simulink model "RedCrane_Control_System_17032025"  (R2024b)
settings: Solver=VariableStepAuto  StartTime=0.0  StopTime=44  RelTol=1e-8
model workspace (MATLAB code in the model file):
  | %% Geometric properties
  | 
  | %Basic geometry width
  | w0 = 0.07;
  | w1 = w0/4;
  | l_RJ = 0.277; %2.1*w0;
  | r_RJ = 0.030;
  | 
  | %Column geometry
  | L_Column = 1.5655; %2;
  | eta_B = -0.25;
  | zeta_B = L_Column;
  | eta_D = -0.365; %0.25;
  | zeta_D = 1.4805; %1.5;
  | eta_J = 0.200; % 0.25;
  | zeta_J = 0.1195; %0.25;
  | 
  | %Column - Main boom link
  | l_DE = 0.490; % 0.5;
  | l_FE = 0.170; % 0.4;
  | 
  | %Main boom geometry
  | L_Mboom = 2.400; % 2;
  | eta_C = 2.400; % 2;
  | zeta_C = 0.070; % 0.25;
  | eta_F = 0.340; % 0.6;
  | zeta_F = 0.010; % -0.25;
  | eta_G = 2.365; % 1.75;
  | zeta_G = 0.235; % -0.25;
  | eta_K = 0.750; % 1;
  | zeta_K = 0.045; % -0.25;
  | 
  | %Main boom-Jib boom link
  | l_GH = 0.490; % 0.5;
  | l_IH = 0.220; % 0.4;
  | 
  | %Jib boom geometry
  | L_Jib_boom = 2.429; % 2;
  | eta_I = 0.280; % 0.5;
  | zeta_I = 0.005; % -0.25;
  | eta_TP = L_Jib_boom;
  | zeta_TP = 0;
  | 
  | % Winch
  | r_W = 0.205/2;
  | L_W = 0.191;
  | eta_W = 0.28722;
  | zeta_W = -0.29926;
  | beta_W = -0.335;
  | 
  | % Mounting plate
  | eta_MP = -0.0249;
  | zeta_MP = -0.17479;
  | beta_MP = 0;
  | 
  | % Pulley
  | r_P = 0.210/2; % Radius pulley
  | eta_P = 2.140;
  | zeta_P = -0.0506;
  | beta_P = -0.0;
  | 
  | %Roller
  | r_RO = 0.055/2; % Radius roller over
  | r_RU = 0.046/2; % Radius roller under
  | eta_RO = 0.306;
  | zeta_RO = 0.12510;
  | 
  | %Mounting
  | L_M = 1; %m
  | W_M = 1; %m
  | H_M = 1; %m
  | eta_M = 0; %m
  | zeta_M = -0.5; %m
  | beta_M = 0; %m
  | 
  | %Ground
  | L_ground = 6; %m
  | W_ground = 4; %m
  | H_ground = 0.01; %m
  | eta_ground = 1.5; %m
  | zeta_ground = -0.5; %m
  | beta_ground = 0; %m
  | 
  | 
  | %% Mass properties (Mass and center of mass)
  | column_mass = 239.4; % kg
  | column_COM = [-0.1007, 0.0001, 0.4351]; % m
  | 
  | MainBoom_mass = 216.5; % kg
  | MainBoom_COM = [1.134, 0.1674, -0.0018]; % m
  | 
  | JibBoom_mass = 842.2; % kg
  | JibBoom_COM = [0.9806, 0.1814, -0.2939]; % m
  | 
  | % Dogbone
  | E2F_mass = 7.076*2; % kg
  | E2F_COM = [0.0817, 0, 0]; % m
  | 
  | D2E_mass = 6.426*2; % kg
  | D2E_COM = [0.245, 0, 0]; % m
  | 
  | G2H_mass = 6.426*2; % kg
  | G2H_COM = [0.245, 0, 0]; % m
  | 
  | H2I_mass = 22.05; % kg
  | H2I_COM = [0.1206, 0, 0]; % m
  | 
  | % Main cylinder
  | MainC_bottom_mass = 57.9561; % kg
  | MainC_bottom_COM = [0.0081, -0.001, 0.4125]; % m
  | 
  | MainC_rod_mass = 43.93; % kg
  | MainC_rod_COM = [0, 0, -0.4290]; % m
  | 
  | % Jib cylinder
  | JibC_bottom_mass = 55.7738; % kg
  | JibC_bottom_COM = [0.0038, 0.0022, 0.4468]; % m
  | 
  | JibC_rod_mass = 45.8854; % kg
  | JibC_rod_COM = [0, 0, -0.4694]; % m
  | 
  | % Winch
  | Winch_mass = 54; % kg
  | Winch_COM = [0, 0, 0]; % m
  | 
  | 
  | %% Inertia properties (Moments of inertia and products of inertia)
  | 
  | column_MOI = [109, 114, 9.009]; % kg*m^2
  | column_POI = [0.0319, -21.59, -0.0113]; % kg*m^2
  | 
  | MainBoom_MOI = [6.5, 160.3, 160]; % kg*m^2
  | MainBoom_POI = [0.0666, 0.1093, 8.016]; % kg*m^2
  | 
  | JibBoom_MOI = [31.75, 566.3, 573.1]; % kg*m^2
  | JibBoom_POI = [-0.0237, -11.42, 9.588]; % kg*m^2
  | 
  | % Dogbone
  | E2F_MOI = [0.0111, 0.0546, 0.0587]; % kg*m^2
  | E2F_POI = [0, -0.0089, 0]; % kg*m^2
  | 
  | D2E_MOI = [0.0069, 0.2419, 0.2485]; % kg*m^2
  | D2E_POI = [0, 0, 0]; % kg*m^2
  | 
  | G2H_MOI = [0.0069, 0.2419, 0.2485]; % kg*m^2
  | G2H_POI = [0, 0, 0]; % kg*m^2
  | 
  | H2I_MOI = [0.2636, 0.4184, 0.1901]; % kg*m^2
  | H2I_POI = [0, 0, 0]; % kg*m^2
  | 
  | 
  | % Main cylinder
  | MainC_bottom_MOI = [7.2059, 7.2304, 0.3979]; % kg*m^2
  | MainC_bottom_POI = [-0.0126, -0.1802, 0.0002]; % kg*m^2
  | 
  | MainC_rod_MOI = [6.0014, 5.9633, 0.1401]; % kg*m^2
  | MainC_rod_POI = [0, -0.0001, 0]; % kg*m^2
  | 
  | % Jib cylinder
  | JibC_bottom_MOI = [8.3780, 8.3476, 0.3607]; % kg*m^2
  | JibC_bottom_POI = [-0.0119, -0.1037, 0.0033]; % kg*m^2
  | 
  | JibC_rod_MOI = [7.4245, 7.3864, 0.1401]; % kg*m^2
  | JibC_rod_POI = [0, -0.0001, 0]; % kg*m^2
  | 
  | % Winch
  | I_W_xx = (1/4)*Winch_mass*r_W^2 + (1/12)*Winch_mass*L_W^2;
  | I_W_yy = (1/4)*Winch_mass*r_W^2 + (1/12)*Winch_mass*L_W^2;
  | I_W_zz = (1/2)*Winch_mass*r_W^2;
  | 
  | Winch_MOI = [I_W_xx, I_W_yy, I_W_zz]; % kg*m^2
  | Winch_POI = [0, 0, 0]; % kg*m^2
  | 
  | 
  | %% Hydraulics
  | 
  | %-------------Cylinder---------------------
  | 
  | % Main cylinder
  | D_piston_MainC = 160; %mm dimater of piston side
  | L_piston_MainC = 65; %66.2;%mm length from joint to buttom of piston side
  | D_rod_MainC = 100; %mm diamter of cylinder rod
  | L_rod_MainC = 978; %990;%mm length from bottom of rod to joint
  | A_piston_MainC = pi/4*D_piston_MainC^2; % mm^2 area of piston side
  | A_rod_MainC = pi/4*D_rod_MainC^2; % mm^2 area of rod
  | A_rodside_MainC = A_piston_MainC-A_rod_MainC; % mm^2 area of rod side
  | L_barrel_MainC = 945-L_piston_MainC; %mm
  | stroke_MainC = 0.75; %m
  | initial_pos_Main = 0.3; %m
  | initial_Pa_Main = 17;%Bar
  | 
  | % Jib cylinder
  | D_piston_JibC = 150; %mm dimater of piston side
  | L_piston_JibC = 65; %66.2;%mm length from joint to buttom of piston side
  | D_rod_JibC = 100; %mm diamter of cylinder rod
  | L_rod_JibC = 1089.5; %1105.5;%mm length from bottom of rod to joint
  | A_piston_JibC = pi/4*D_piston_JibC^2; % mm^2 area of piston side
  | A_rod_JibC = pi/4*D_rod_JibC^2; % mm^2 area of rod
  | A_rodside_JibC = A_piston_JibC-A_rod_JibC; % mm^2 area of rod side
  | L_barrel_JibC = 1050-L_piston_JibC; %mm
  | stroke_JibC = 0.855; %m
  | initial_pos_Jib = 0.855; %m
  | initial_Pa_Jib = 1;%Bar
  | initial_Pb_Jib = 67;%Bar
  | 
  | % winch
  | poly_b = [1.762740809095876e+02,-44.442169999547330];
  | poly_c = [1.901177983521692e+02,-1.484122102902541e+02];
  | angle_b = poly_b(1)*initial_pos_Main + poly_b(2);
  | angle_c = poly_c(1)*initial_pos_Jib + poly_c(2);
  | angle_w = -90 - angle_c - angle_b;
  | 
  | %Motor
  | DM = 200; %Displacement cm^3/rev
  | GR = 5.04; % Gear ratio 1:5,04
  | 
  | 
  | % ------------------CBV-------------------
  | 
  | % Main
  | pCr_Main = 43.95;%Bar
  | dp_open_Main = 124.43;%Bar
  | 
  | % Jib
  | alpha = 2.7;
  | pCr_Jib_A = 320;%Bar
  | dp_open_Jib_A = 65;%Bar
  | pCr_Jib_B = 280;%Bar
  | dp_open_Jib_B = 40;%Bar
  | 
  | %-------------------DCV-----------------------
  | Cd = 0.64;
  | Q_rat = 30/6e4;
  | dp_2 = 6e5;
  | dp_1 = 1e5;
  | roh = 850;
  | 
  | % Main dcv
  | dead_up_Main = 0.071;
  | dead_down_Main = 0.126;
  | 
  | % Jib dcv
  | dead_up_Jib = 0.037;
  | dead_down_Jib = 0.126;
  | 
  | Ad2 = Q_rat/(Cd*sqrt(2/roh*dp_2))*1e6; %mm
  | Ad1_1 = Q_rat/(Cd*sqrt(2/roh*dp_1))*1e6;
  | Ad1_0 = Q_rat/(Cd*sqrt(2/roh*dp_1))*1e6*0;
  | 
  | Ad1_Main_up = Q_rat/(Cd*sqrt(2/roh*dp_1))*1e6*dead_up_Main;
  | Ad1_Main_down = Q_rat/(Cd*sqrt(2/roh*dp_1))*1e6*dead_down_Main;
  | Ad1_Jib_up = Q_rat/(Cd*sqrt(2/roh*dp_1))*1e6*dead_up_Jib;
  | Ad1_Jib_down = Q_rat/(Cd*sqrt(2/roh*dp_1))*1e6*dead_down_Jib;
undefined symbols (not defined in the file or in its folder): dead_down_m, dead_up_m, X, Y, Z
libraries: sm_lib x171, fl_lib x94, nesl_utility x64, SimscapeFluids_lib x33, sdl_lib x1
(part 5 of 9)

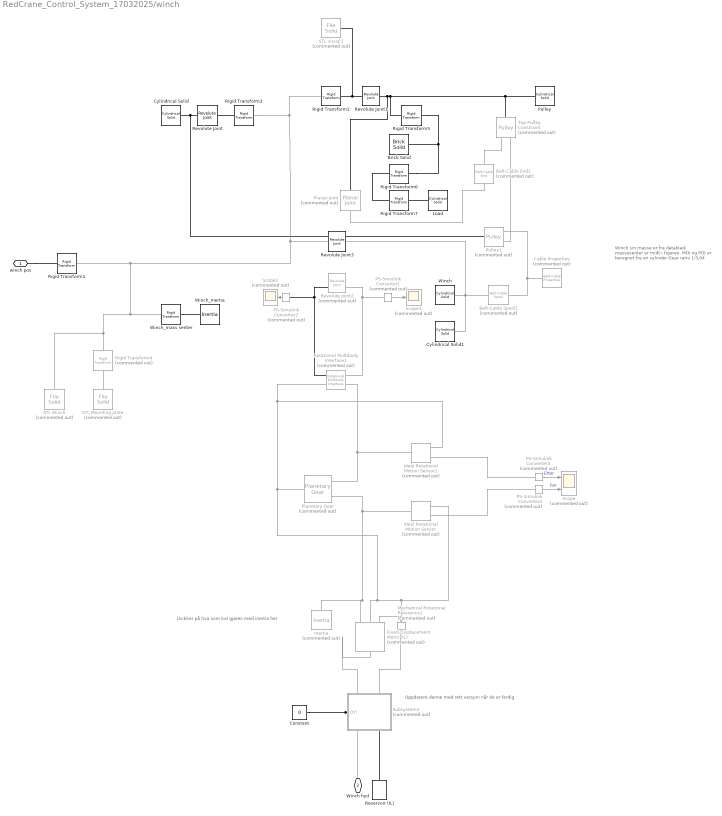
== system RedCrane_Control_System_17032025/winch ==
  note: Oppdatere denne med rett versjon når de er
      | ferdig
  note: Winch sin masse er fra datablad,
      | massesenter er midt i figuren.
      |
      | MOI og POI er beregnet fra en
      | sylinder
      |
      | Gear ratio 1:5,04
  note: Usikker på hva som kal gjøres med inertia her
  Belt-Cable End2 : sm_lib/Belts and Cables/Belt-Cable End  Commented=on
  Belt-Cable Spool1 : sm_lib/Belts and Cables/Belt-Cable Spool  Commented=on  PitchRadius=r_W  PitchRadiusUnits=m  SenseSpoolAngleA=off  SenseFleetAngleA=off
  Brick Solid : sm_lib/Body Elements/Brick Solid  BrickDimensions=[1 0.01 0.01]  BrickDimensionsUnits=m  ExportEntireGeometry=off  InertiaType=CalculateFromGeometry  BasedOnType=Density  Density=0  DensityUnits=kg/m^3  Mass=1  MassUnits=kg  CenterOfMass=[0 0 0]  CenterOfMassUnits=m  MomentsOfInertia=[1 1 1]  MomentsOfInertiaUnits=kg*m^2  ProductsOfInertia=[0 0 0]  ProductsOfInertiaUnits=kg*m^2  GraphicType=FromGeometry  MarkerShape=Sphere  MarkerSize=10  GraphicVisPropType=SimpleVisualProperties  GraphicDiffuseColor=[0.5 0.5 0.5]  GraphicOpacity=1  GraphicSpecularColor=[0.5 0.5 0.5 1.0]  GraphicAmbientColor=[0.15 0.15 0.15 1.0]  GraphicEmissiveColor=[0.0 0.0 0.0 1.0]  GraphicShininess=75  DoExposeReferenceFrame=on  SerializedFrames=<Frames/>
  Cable Properties : sm_lib/Belts and Cables/Belt-Cable Properties  Commented=on  DrumBeltCableAlignment=Unrestricted  GraphicType=PitchLine  GraphicVisPropType=SimpleVisualProperties  GraphicDiffuseColor=[0.4 0.0 1.0]  GraphicOpacity=1.0  GraphicSpecularColor=[0.5 0.5 0.5 1.0]  GraphicAmbientColor=[0.15 0.15 0.15 1.0]  GraphicEmissiveColor=[0.0 0.0 0.0 1.0]  GraphicShininess=75
  Constant : Constant  Value=0
  Cylindrical Solid : sm_lib/Body Elements/Cylindrical Solid  CylinderRadius=r_RO  CylinderRadiusUnits=m  CylinderLength=L_W  CylinderLengthUnits=m  ExportEntireGeometry=off  InertiaType=Custom  BasedOnType=Density  Density=1000  DensityUnits=kg/m^3  Mass=1  MassUnits=kg  CenterOfMass=[0 0 0]  CenterOfMassUnits=m  MomentsOfInertia=[1 1 1]  MomentsOfInertiaUnits=kg*m^2  ProductsOfInertia=[0 0 0]  ProductsOfInertiaUnits=kg*m^2  GraphicType=FromGeometry  MarkerShape=Sphere  MarkerSize=10  GraphicVisPropType=SimpleVisualProperties  GraphicDiffuseColor=[1 1 1]  GraphicOpacity=1  GraphicSpecularColor=[0.5 0.5 0.5 1.0]  GraphicAmbientColor=[0.15 0.15 0.15 1.0]  GraphicEmissiveColor=[0.0 0.0 0.0 1.0]  GraphicShininess=75  DoExposeReferenceFrame=on  SerializedFrames=<Frames/>
  Cylindrical Solid1 : sm_lib/Body Elements/Cylindrical Solid  CylinderRadius=(305-10.5)/2  CylinderRadiusUnits=mm  CylinderLength=0.2  CylinderLengthUnits=m  ExportEntireGeometry=off  InertiaType=PointMass  BasedOnType=Density  Density=1000  DensityUnits=kg/m^3  Mass=279.7880-50  MassUnits=kg  CenterOfMass=[0 0 0]  CenterOfMassUnits=m  MomentsOfInertia=[1 1 1]  MomentsOfInertiaUnits=kg*m^2  ProductsOfInertia=[0 0 0]  ProductsOfInertiaUnits=kg*m^2  GraphicType=FromGeometry  MarkerShape=Sphere  MarkerSize=10  GraphicVisPropType=SimpleVisualProperties  GraphicDiffuseColor=[0.902 0.902 0.902]  GraphicOpacity=1  GraphicSpecularColor=[0.5 0.5 0.5 1.0]  GraphicAmbientColor=[0.15 0.15 0.15 1.0]  GraphicEmissiveColor=[0.0 0.0 0.0 1.0]  GraphicShininess=75  DoExposeReferenceFrame=on  SerializedFrames=<Frames/>
  Fixed-Displacement Motor (IL) : SimscapeFluids_lib/Isothermal Liquid/Pumps & Motors/Fixed-Displacement Motor (IL)  Commented=on  leakage_friction_spec=fluids.isothermal_liquid.pumps_motors.enum.MotorLossSpec.Analytical  displacement=DM cm^3/rev  omega_nominal=1800 rpm  p_nominal=10 MPa  vol_eff_nominal=1  mech_eff_nominal=1  no_load_torque=0 N*m  p_diff_eff_TLU=[.1, 1, 2] MPa  omega_eff_TLU=[250, 500, 1000, 2000, 3000, 4000] rpm  vol_eff_TLU=[.816, .908, .954, .977, .981, .984; .325, .663, .831, .916, .925, .946; .137, .568, .78, .892, .893, .91]  mech_eff_TLU=[.996, .996, .996, .996, .996, .996; .988, .989, .989, .989, .989, .99; .981, .981, .982, .982, .983, .984]  p_diff_loss_TLU=[.1, 1, 2] MPa  omega_loss_TLU=[250, 500, 1000, 2000, 3000, 4000] rpm  vol_loss_TLU=1e-3 * [.023, .023, .023, .023, .0285, .032; .0844, .0842, .0845, .084, .1125, .108; .1079, .108, .11, .108, .1605, .18] m^3/s  mech_loss_TLU=[.002, .002, .002, .002, .002, .002; .0607, .0556, .0556, .0556, .0556, .0505; .1937, .1937, .1833, .1833, .1729, .1626] N*m  q_shaft_TLU=[.125, .25, .5, 1, 1.5, 2] * 1e-3 m^3/s  p_diff_shaft_TLU=[.1, 1, 2] MPa  torque_shaft_TLU=[.47, 4.72, 9.35; .47, 4.7, 9.36; .47, 4.7, 9.4; .47, 4.7, 9.41; .47, 4.7, 9.46; .47, 4.68, 9.5] N*m  omega_shaft_TLU=[205, 80, 35; 455, 330, 285; 955, 831, 780; 1950, 1830, 1780; 2940, 2775, 2680; 3940, 3780, 3640] rpm  vol_eff_min=1e-3  vol_eff_max=1  mech_eff_min=1e-3  mech_eff_max=1  pressure_threshold=1e-3 MPa  omega_threshold=100 rpm  supplied_range_check=simscape.enum.assert.action.none  motor_mode_check=simscape.enum.assert.action.none  pressure_check=simscape.enum.assert.action.none  p_min_valid=0.101325 MPa
      settings: InternalSimscapePortConfiguration="{\"Bottom\":[{\"id\":\"B\",\"label\":\"B\",\"type\":\"foundation.isothermal_liquid.isothermal_liquid\"}],\"Left\":[],\"Right\":[{\"id\":\"R\",\"label\":\"R\",\"type\":\"foundation.mechanical.rotational.rotational\"},{\"id\":\"C\",\"label\":\"C\",\"type\":\"foundation.mechanical.rotational.rotational\"}],\"Top\":[{\"id\":\"A\",\"label\":\"A\",\"type\":\"foundation.isothermal_liquid.isothermal_liquid\"}]}"
  Ideal Rotational Motion Sensor : fl_lib/Mechanical/Mechanical Sensors/Ideal Rotational Motion Sensor  Commented=on  reference=foundation.enum.MeasurementReference.difference  acceleration_port=false  velocity_port=true  position_port=false  wrap_angle=false  offset=0 rad
      settings: InternalSimscapePortConfiguration="{\"Bottom\":[],\"Left\":[{\"id\":\"R\",\"label\":\"R\",\"type\":\"foundation.mechanical.rotational.rotational\"}],\"Right\":[{\"id\":\"C\",\"label\":\"C\",\"type\":\"foundation.mechanical.rotational.rotational\"},{\"id\":\"W\",\"label\":\"W\",\"type\":\"output\"}],\"Top\":[]}"
  Ideal Rotational Motion Sensor1 : fl_lib/Mechanical/Mechanical Sensors/Ideal Rotational Motion Sensor  Commented=on  reference=foundation.enum.MeasurementReference.difference  acceleration_port=false  velocity_port=true  position_port=false  wrap_angle=false  offset=0 rad
      settings: InternalSimscapePortConfiguration="{\"Bottom\":[],\"Left\":[{\"id\":\"R\",\"label\":\"R\",\"type\":\"foundation.mechanical.rotational.rotational\"}],\"Right\":[{\"id\":\"C\",\"label\":\"C\",\"type\":\"foundation.mechanical.rotational.rotational\"},{\"id\":\"W\",\"label\":\"W\",\"type\":\"output\"}],\"Top\":[]}"
  Inertia : fl_lib/Mechanical/Rotational Elements/Inertia  Commented=on  inertia=0.01 kg*m^2  num_ports=foundation.enum.numPorts2.one  w_specify=off  w_priority=High  w=0 rad/s  w_nominal_specify=off  w_nominal_value=1  w_nominal_unit=rad/s  t_specify=off  t_priority=None  t=0 N*m  t_nominal_specify=off  t_nominal_value=1  t_nominal_unit=N*m
  Load : sm_lib/Body Elements/Cylindrical Solid  CylinderRadius=81/2  CylinderRadiusUnits=mm  CylinderLength=240  CylinderLengthUnits=mm  ExportEntireGeometry=off  InertiaType=CalculateFromGeometry  BasedOnType=Mass  Density=1000  DensityUnits=kg/m^3  Mass=10  MassUnits=kg  CenterOfMass=[0 0 0]  CenterOfMassUnits=m  MomentsOfInertia=[1 1 1]  MomentsOfInertiaUnits=kg*m^2  ProductsOfInertia=[0 0 0]  ProductsOfInertiaUnits=kg*m^2  GraphicType=FromGeometry  MarkerShape=Sphere  MarkerSize=10  GraphicVisPropType=SimpleVisualProperties  GraphicDiffuseColor=[0.9412 0.9412 0.07451]  GraphicOpacity=1  GraphicSpecularColor=[0.5 0.5 0.5 1.0]  GraphicAmbientColor=[0.15 0.15 0.15 1.0]  GraphicEmissiveColor=[0.0 0.0 0.0 1.0]  GraphicShininess=75  DoExposeReferenceFrame=on  SerializedFrames=<Frames/>
  Mechanical Rotational Reference1 : fl_lib/Mechanical/Rotational Elements/Mechanical Rotational Reference  Commented=on
  PS-Simulink Converter{1..4} (4 alike) : nesl_utility/PS-Simulink Converter  Commented=on  PhysicalDomain=network_engine_domain  SubClassName=ps_output  LeftPortType=input  RightPortType=output  PseudoPeriodic=off  Frequencies=[]  VectorFormat=inherit  Unit=inherit  AffineConversion=off
  Planar Joint : sm_lib/Joints/Planar Joint  Commented=on  JointMode=Normal  CompositeWrenchDir=FollowerOnBase  CompositeWrenchFrame=BaseFrame  SenseConstraintForce=off  SenseConstraintTorque=off  SenseTotalForce=off  SenseTotalTorque=off  PxPositionTargetSpecify=on  PxPositionTargetPriority=High  PxPositionTargetValue=1  PxPositionTargetValueUnits=m  PxVelocityTargetSpecify=off  PxVelocityTargetPriority=High  PxVelocityTargetValue=0  PxVelocityTargetValueUnits=m/s  PxEquilibriumPosition=0  PxEquilibriumPositionUnits=m  PxSpringStiffness=0  PxSpringStiffnessUnits=N/m  PxDampingCoefficient=1e-1  PxDampingCoefficientUnits=N/(m/s)  PxLowerLimitSpecify=off  PxLowerLimitBound=-1  PxLowerLimitBoundUnits=m  PxLowerLimitStiffness=1e6  PxLowerLimitStiffnessUnits=N/m  PxLowerLimitDamping=1e3  PxLowerLimitDampingUnits=N/(m/s)  PxLowerLimitTransitionRegionWidth=1e-4  PxLowerLimitTransitionRegionWidthUnits=m  PxUpperLimitSpecify=off  PxUpperLimitBound=1  PxUpperLimitBoundUnits=m  PxUpperLimitStiffness=1e6  PxUpperLimitStiffnessUnits=N/m  PxUpperLimitDamping=1e3  PxUpperLimitDampingUnits=N/(m/s)  PxUpperLimitTransitionRegionWidth=1e-4  PxUpperLimitTransitionRegionWidthUnits=m  PxTorqueActuationMode=NoTorque  PxMotionActuationMode=ComputedMotion  PxSensePosition=off  PxSenseVelocity=off  PxSenseAcceleration=off  PxSenseTorqueForce=off  PxSenseLowerLimitTorqueForce=off  PxSenseUpperLimitTorqueForce=off  PyPositionTargetSpecify=on  PyPositionTargetPriority=High  PyPositionTargetValue=r_P  PyPositionTargetValueUnits=m  PyVelocityTargetSpecify=off  PyVelocityTargetPriority=High  PyVelocityTargetValue=0  PyVelocityTargetValueUnits=m/s  PyEquilibriumPosition=0  PyEquilibriumPositionUnits=m  PySpringStiffness=0  PySpringStiffnessUnits=N/m  PyDampingCoefficient=1e-1  PyDampingCoefficientUnits=N/(m/s)  PyLowerLimitSpecify=off  PyLowerLimitBound=-1  PyLowerLimitBoundUnits=m  PyLowerLimitStiffness=1e6  PyLowerLimitStiffnessUnits=N/m  PyLowerLimitDamping=1e3  PyLowerLimitDampingUnits=N/(m/s)  PyLowerLimitTransitionRegionWidth=1e-4  PyLowerLimitTransitionRegionWidthUnits=m  PyUpperLimitSpecify=off  PyUpperLimitBound=1  PyUpperLimitBoundUnits=m  PyUpperLimitStiffness=1e6  PyUpperLimitStiffnessUnits=N/m  PyUpperLimitDamping=1e3  PyUpperLimitDampingUnits=N/(m/s)  PyUpperLimitTransitionRegionWidth=1e-4  PyUpperLimitTransitionRegionWidthUnits=m  PyTorqueActuationMode=NoTorque  PyMotionActuationMode=ComputedMotion  PySensePosition=off  PySenseVelocity=off  PySenseAcceleration=off  PySenseTorqueForce=off  PySenseLowerLimitTorqueForce=off  PySenseUpperLimitTorqueForce=off  RzPositionTargetSpecify=off  RzPositionTargetPriority=High  RzPositionTargetValue=90  RzPositionTargetValueUnits=deg  RzVelocityTargetSpecify=off  RzVelocityTargetPriority=High  RzVelocityTargetValue=0  RzVelocityTargetValueUnits=deg/s  RzEquilibriumPosition=0  RzEquilibriumPositionUnits=deg  RzSpringStiffness=0  RzSpringStiffnessUnits=N*m/deg  RzDampingCoefficient=0  RzDampingCoefficientUnits=N*m/(deg/s)  RzLowerLimitSpecify=off  RzLowerLimitBound=-90  RzLowerLimitBoundUnits=deg  RzLowerLimitStiffness=1e4  RzLowerLimitStiffnessUnits=N*m/deg  RzLowerLimitDamping=10  RzLowerLimitDampingUnits=N*m/(deg/s)  RzLowerLimitTransitionRegionWidth=0.1  RzLowerLimitTransitionRegionWidthUnits=deg  RzUpperLimitSpecify=off  RzUpperLimitBound=90  RzUpperLimitBoundUnits=deg  RzUpperLimitStiffness=1e4  RzUpperLimitStiffnessUnits=N*m/deg  RzUpperLimitDamping=10  RzUpperLimitDampingUnits=N*m/(deg/s)  RzUpperLimitTransitionRegionWidth=0.1  RzUpperLimitTransitionRegionWidthUnits=deg  RzTorqueActuationMode=NoTorque  RzMotionActuationMode=ComputedMotion  RzSensePosition=off  RzSenseVelocity=off  RzSenseAcceleration=off  RzSenseTorqueForce=off  RzSenseLowerLimitTorqueForce=off  RzSenseUpperLimitTorqueForce=off
  Planetary Gear : sdl_lib/Gears/Planetary Gear  Commented=on  rs_ratio=GR  friction_model=sdl.enum.gear_friction.none  efficiency=[.96, .98]  temperature_TLU=[280, 300, 320] K  efficiency_sp_TLU=[.95, .9, .85]  efficiency_rp_TLU=[.95, .9, .85]  pwr_thr=[.001, .001] W  mu_visc=[0, 0] N*m*s/rad  model_inertia=simscape.enum.onoff.off  sun_inertia=0.001 kg*m^2  ring_inertia=0.001 kg*m^2  carrier_inertia=0.001 kg*m^2  carrier_radius=0.01 m  planet_inertia=0.001 kg*m^2  planet_mass=0.001 kg  thermal_mass=50 J/K  T_init=300 K
  Pulley : sm_lib/Body Elements/Cylindrical Solid  CylinderRadius=r_P  CylinderRadiusUnits=m  CylinderLength=L_W  CylinderLengthUnits=m  ExportEntireGeometry=off  InertiaType=Custom  BasedOnType=Density  Density=1000  DensityUnits=kg/m^3  Mass=1  MassUnits=kg  CenterOfMass=[0 0 0]  CenterOfMassUnits=m  MomentsOfInertia=[1 1 1]  MomentsOfInertiaUnits=kg*m^2  ProductsOfInertia=[0 0 0]  ProductsOfInertiaUnits=kg*m^2  GraphicType=FromGeometry  MarkerShape=Sphere  MarkerSize=10  GraphicVisPropType=SimpleVisualProperties  GraphicDiffuseColor=[0.149 0.149 0.149]  GraphicOpacity=1  GraphicSpecularColor=[0.5 0.5 0.5 1.0]  GraphicAmbientColor=[0.15 0.15 0.15 1.0]  GraphicEmissiveColor=[0.0 0.0 0.0 1.0]  GraphicShininess=75  DoExposeReferenceFrame=on  SerializedFrames=<Frames/>
  Pulley1 : sm_lib/Belts and Cables/Pulley  Commented=on  PitchRadius=r_RO  PitchRadiusUnits=m  InitialWrapAngleLowerBound=0  InitialWrapAngleLowerBoundUnits=deg  SenseWrapAngle=off  SensePulleyAngleA=off  SensePulleyAngleB=off  SenseFleetAngleA=off  SenseFleetAngleB=off
  Reservoir (IL) : fl_lib/Isothermal Liquid/Elements/Reservoir (IL)  reservoir_type=foundation.enum.constant_controlled.constant  pressure_spec=foundation.enum.pressure_spec.atmospheric  reservoir_pressure=0.101325 MPa
  Revolute Joint : sm_lib/Joints/Revolute Joint  JointMode=Normal  CompositeWrenchDir=FollowerOnBase  CompositeWrenchFrame=BaseFrame  SenseConstraintForce=off  SenseConstraintTorque=off  SenseTotalForce=off  SenseTotalTorque=off  PositionTargetSpecify=off  PositionTargetPriority=High  PositionTargetValue=0  PositionTargetValueUnits=deg  VelocityTargetSpecify=off  VelocityTargetPriority=High  VelocityTargetValue=0  VelocityTargetValueUnits=deg/s  EquilibriumPosition=0  EquilibriumPositionUnits=deg  SpringStiffness=0  SpringStiffnessUnits=N*m/deg  DampingCoefficient=0  DampingCoefficientUnits=N*m/(deg/s)  LowerLimitSpecify=off  LowerLimitBound=-90  LowerLimitBoundUnits=deg  LowerLimitStiffness=1e4  LowerLimitStiffnessUnits=N*m/deg  LowerLimitDamping=10  LowerLimitDampingUnits=N*m/(deg/s)  LowerLimitTransitionRegionWidth=0.1  LowerLimitTransitionRegionWidthUnits=deg  UpperLimitSpecify=off  UpperLimitBound=90  UpperLimitBoundUnits=deg  UpperLimitStiffness=1e4  UpperLimitStiffnessUnits=N*m/deg  UpperLimitDamping=10  UpperLimitDampingUnits=N*m/(deg/s)  UpperLimitTransitionRegionWidth=0.1  UpperLimitTransitionRegionWidthUnits=deg  TorqueActuationMode=NoTorque  MotionActuationMode=ComputedMotion  SensePosition=off  SenseVelocity=off  SenseAcceleration=off  SenseTorqueForce=off  SenseLowerLimitTorqueForce=off  SenseUpperLimitTorqueForce=off
  Revolute Joint1 : sm_lib/Joints/Revolute Joint  JointMode=Normal  CompositeWrenchDir=FollowerOnBase  CompositeWrenchFrame=BaseFrame  SenseConstraintForce=off  SenseConstraintTorque=off  SenseTotalForce=off  SenseTotalTorque=off  PositionTargetSpecify=on  PositionTargetPriority=High  PositionTargetValue=angle_w  PositionTargetValueUnits=deg  VelocityTargetSpecify=on  VelocityTargetPriority=High  VelocityTargetValue=0  VelocityTargetValueUnits=deg/s  EquilibriumPosition=0  EquilibriumPositionUnits=deg  SpringStiffness=0  SpringStiffnessUnits=N*m/deg  DampingCoefficient=0  DampingCoefficientUnits=N*m/(deg/s)  LowerLimitSpecify=off  LowerLimitBound=-90  LowerLimitBoundUnits=deg  LowerLimitStiffness=1e4  LowerLimitStiffnessUnits=N*m/deg  LowerLimitDamping=10  LowerLimitDampingUnits=N*m/(deg/s)  LowerLimitTransitionRegionWidth=0.1  LowerLimitTransitionRegionWidthUnits=deg  UpperLimitSpecify=off  UpperLimitBound=90  UpperLimitBoundUnits=deg  UpperLimitStiffness=1e4  UpperLimitStiffnessUnits=N*m/deg  UpperLimitDamping=10  UpperLimitDampingUnits=N*m/(deg/s)  UpperLimitTransitionRegionWidth=0.1  UpperLimitTransitionRegionWidthUnits=deg  TorqueActuationMode=NoTorque  MotionActuationMode=ComputedMotion  SensePosition=off  SenseVelocity=off  SenseAcceleration=off  SenseTorqueForce=off  SenseLowerLimitTorqueForce=off  SenseUpperLimitTorqueForce=off
  Revolute Joint2 : sm_lib/Joints/Revolute Joint  Commented=on  JointMode=Normal  CompositeWrenchDir=FollowerOnBase  CompositeWrenchFrame=BaseFrame  SenseConstraintForce=off  SenseConstraintTorque=off  SenseTotalForce=off  SenseTotalTorque=off  PositionTargetSpecify=on  PositionTargetPriority=High  PositionTargetValue=0  PositionTargetValueUnits=deg  VelocityTargetSpecify=on  VelocityTargetPriority=High  VelocityTargetValue=0  VelocityTargetValueUnits=deg/s  EquilibriumPosition=0  EquilibriumPositionUnits=deg  SpringStiffness=0  SpringStiffnessUnits=N*m/deg  DampingCoefficient=0  DampingCoefficientUnits=N*m/(deg/s)  LowerLimitSpecify=off  LowerLimitBound=-90  LowerLimitBoundUnits=deg  LowerLimitStiffness=1e4  LowerLimitStiffnessUnits=N*m/deg  LowerLimitDamping=10  LowerLimitDampingUnits=N*m/(deg/s)  LowerLimitTransitionRegionWidth=0.1  LowerLimitTransitionRegionWidthUnits=deg  UpperLimitSpecify=off  UpperLimitBound=90  UpperLimitBoundUnits=deg  UpperLimitStiffness=1e4  UpperLimitStiffnessUnits=N*m/deg  UpperLimitDamping=10  UpperLimitDampingUnits=N*m/(deg/s)  UpperLimitTransitionRegionWidth=0.1  UpperLimitTransitionRegionWidthUnits=deg  TorqueActuationMode=InputTorque  MotionActuationMode=ComputedMotion  SensePosition=off  SenseVelocity=on  SenseAcceleration=off  SenseTorqueForce=off  SenseLowerLimitTorqueForce=off  SenseUpperLimitTorqueForce=off
  Revolute Joint3 : sm_lib/Joints/Revolute Joint  JointMode=Locked  CompositeWrenchDir=FollowerOnBase  CompositeWrenchFrame=BaseFrame  SenseConstraintForce=off  SenseConstraintTorque=off  SenseTotalForce=off  SenseTotalTorque=off  PositionTargetSpecify=on  PositionTargetPriority=High  PositionTargetValue=0  PositionTargetValueUnits=deg  VelocityTargetSpecify=on  VelocityTargetPriority=High  VelocityTargetValue=0  VelocityTargetValueUnits=deg/s  EquilibriumPosition=0  EquilibriumPositionUnits=deg  SpringStiffness=0  SpringStiffnessUnits=N*m/deg  DampingCoefficient=0  DampingCoefficientUnits=N*m/(deg/s)  LowerLimitSpecify=off  LowerLimitBound=-90  LowerLimitBoundUnits=deg  LowerLimitStiffness=1e4  LowerLimitStiffnessUnits=N*m/deg  LowerLimitDamping=10  LowerLimitDampingUnits=N*m/(deg/s)  LowerLimitTransitionRegionWidth=0.1  LowerLimitTransitionRegionWidthUnits=deg  UpperLimitSpecify=off  UpperLimitBound=90  UpperLimitBoundUnits=deg  UpperLimitStiffness=1e4  UpperLimitStiffnessUnits=N*m/deg  UpperLimitDamping=10  UpperLimitDampingUnits=N*m/(deg/s)  UpperLimitTransitionRegionWidth=0.1  UpperLimitTransitionRegionWidthUnits=deg  TorqueActuationMode=NoTorque  MotionActuationMode=ComputedMotion  SensePosition=off  SenseVelocity=off  SenseAcceleration=off  SenseTorqueForce=off  SenseLowerLimitTorqueForce=off  SenseUpperLimitTorqueForce=off
  Rigid Transform1 : sm_lib/Frames and Transforms/Rigid Transform  RotationMethod=None  FollAlignAxisA=+X  BaseAlignAxisA=+Y  FollAlignAxisB=+Y  BaseAlignAxisB=+Z  RotationStandardAxis=+Z  RotationAngle=0  RotationAngleUnits=deg  RotationArbitraryAxis=[0 0 1]  RotationSequenceAxes=FollowerAxes  RotationSequence=XYZ  RotationSequenceAngles=[90 0 0]  RotationSequenceAnglesUnits=deg  RotationMatrix=[1 0 0;0 1 0;0 0 1]  Quaternion=[1 0 0 0]  TranslationMethod=Cartesian  TranslationCartesianOffset=[eta_W zeta_W beta_W]  TranslationCartesianOffsetUnits=m  TranslationStandardAxis=+Z  TranslationStandardOffset=0  TranslationStandardOffsetUnits=m  TranslationROffset=0  TranslationROffsetUnits=m  TranslationThetaOffset=0  TranslationThetaOffsetUnits=deg  TranslationZOffset=0  TranslationZOffsetUnits=m
  Rigid Transform2 : sm_lib/Frames and Transforms/Rigid Transform  RotationMethod=None  FollAlignAxisA=+X  BaseAlignAxisA=+Y  FollAlignAxisB=+Y  BaseAlignAxisB=+Z  RotationStandardAxis=+X  RotationAngle=90  RotationAngleUnits=deg  RotationArbitraryAxis=[0 0 1]  RotationSequenceAxes=FollowerAxes  RotationSequence=XYX  RotationSequenceAngles=[0 0 0]  RotationSequenceAnglesUnits=deg  RotationMatrix=[1 0 0;0 1 0;0 0 1]  Quaternion=[1 0 0 0]  TranslationMethod=Cartesian  TranslationCartesianOffset=[eta_P zeta_P beta_P]  TranslationCartesianOffsetUnits=m  TranslationStandardAxis=+Z  TranslationStandardOffset=0  TranslationStandardOffsetUnits=m  TranslationROffset=0  TranslationROffsetUnits=m  TranslationThetaOffset=0  TranslationThetaOffsetUnits=deg  TranslationZOffset=0  TranslationZOffsetUnits=m
  Rigid Transform3 : sm_lib/Frames and Transforms/Rigid Transform  RotationMethod=None  FollAlignAxisA=+X  BaseAlignAxisA=+Y  FollAlignAxisB=+Y  BaseAlignAxisB=+Z  RotationStandardAxis=+X  RotationAngle=90  RotationAngleUnits=deg  RotationArbitraryAxis=[0 0 1]  RotationSequenceAxes=FollowerAxes  RotationSequence=XYX  RotationSequenceAngles=[0 0 0]  RotationSequenceAnglesUnits=deg  RotationMatrix=[1 0 0;0 1 0;0 0 1]  Quaternion=[1 0 0 0]  TranslationMethod=Cartesian  TranslationCartesianOffset=[eta_RO zeta_RO 0]  TranslationCartesianOffsetUnits=m  TranslationStandardAxis=+Z  TranslationStandardOffset=0  TranslationStandardOffsetUnits=m  TranslationROffset=0  TranslationROffsetUnits=m  TranslationThetaOffset=0  TranslationThetaOffsetUnits=deg  TranslationZOffset=0  TranslationZOffsetUnits=m
  Rigid Transform4 : sm_lib/Frames and Transforms/Rigid Transform  Commented=on  RotationMethod=None  FollAlignAxisA=+X  BaseAlignAxisA=+Y  FollAlignAxisB=+Y  BaseAlignAxisB=+Z  RotationStandardAxis=-X  RotationAngle=90  RotationAngleUnits=deg  RotationArbitraryAxis=[0 0 1]  RotationSequenceAxes=FollowerAxes  RotationSequence=XYX  RotationSequenceAngles=[0 0 0]  RotationSequenceAnglesUnits=deg  RotationMatrix=[1 0 0;0 1 0;0 0 1]  Quaternion=[1 0 0 0]  TranslationMethod=Cartesian  TranslationCartesianOffset=[eta_MP zeta_MP beta_MP]  TranslationCartesianOffsetUnits=m  TranslationStandardAxis=+Z  TranslationStandardOffset=0  TranslationStandardOffsetUnits=m  TranslationROffset=0  TranslationROffsetUnits=m  TranslationThetaOffset=0  TranslationThetaOffsetUnits=deg  TranslationZOffset=0  TranslationZOffsetUnits=m
  Rigid Transform5 : sm_lib/Frames and Transforms/Rigid Transform  RotationMethod=None  FollAlignAxisA=+X  BaseAlignAxisA=+Y  FollAlignAxisB=+Y  BaseAlignAxisB=+Z  RotationStandardAxis=+X  RotationAngle=90  RotationAngleUnits=deg  RotationArbitraryAxis=[0 0 1]  RotationSequenceAxes=FollowerAxes  RotationSequence=XYX  RotationSequenceAngles=[0 0 0]  RotationSequenceAnglesUnits=deg  RotationMatrix=[1 0 0;0 1 0;0 0 1]  Quaternion=[1 0 0 0]  TranslationMethod=Cartesian  TranslationCartesianOffset=[0.5 , 0, 0]  TranslationCartesianOffsetUnits=m  TranslationStandardAxis=+Z  TranslationStandardOffset=0  TranslationStandardOffsetUnits=m  TranslationROffset=0  TranslationROffsetUnits=m  TranslationThetaOffset=0  TranslationThetaOffsetUnits=deg  TranslationZOffset=0  TranslationZOffsetUnits=m
  Rigid Transform6 : sm_lib/Frames and Transforms/Rigid Transform  RotationMethod=None  FollAlignAxisA=+X  BaseAlignAxisA=+Y  FollAlignAxisB=+Y  BaseAlignAxisB=+Z  RotationStandardAxis=+X  RotationAngle=90  RotationAngleUnits=deg  RotationArbitraryAxis=[0 0 1]  RotationSequenceAxes=FollowerAxes  RotationSequence=XYX  RotationSequenceAngles=[0 0 0]  RotationSequenceAnglesUnits=deg  RotationMatrix=[1 0 0;0 1 0;0 0 1]  Quaternion=[1 0 0 0]  TranslationMethod=Cartesian  TranslationCartesianOffset=[0.5 , 0, 0]  TranslationCartesianOffsetUnits=m  TranslationStandardAxis=+Z  TranslationStandardOffset=0  TranslationStandardOffsetUnits=m  TranslationROffset=0  TranslationROffsetUnits=m  TranslationThetaOffset=0  TranslationThetaOffsetUnits=deg  TranslationZOffset=0  TranslationZOffsetUnits=m
  Rigid Transform7 : sm_lib/Frames and Transforms/Rigid Transform  RotationMethod=StandardAxis  FollAlignAxisA=+X  BaseAlignAxisA=+Y  FollAlignAxisB=+Y  BaseAlignAxisB=+Z  RotationStandardAxis=+Y  RotationAngle=90  RotationAngleUnits=deg  RotationArbitraryAxis=[0 0 1]  RotationSequenceAxes=FollowerAxes  RotationSequence=XYX  RotationSequenceAngles=[0 0 0]  RotationSequenceAnglesUnits=deg  RotationMatrix=[1 0 0;0 1 0;0 0 1]  Quaternion=[1 0 0 0]  TranslationMethod=None  TranslationCartesianOffset=[0.5 , 0, 0]  TranslationCartesianOffsetUnits=m  TranslationStandardAxis=+Z  TranslationStandardOffset=0  TranslationStandardOffsetUnits=m  TranslationROffset=0  TranslationROffsetUnits=m  TranslationThetaOffset=0  TranslationThetaOffsetUnits=deg  TranslationZOffset=0  TranslationZOffsetUnits=m
  Rotational Multibody Interface1 : fl_lib/Mechanical/Multibody Interfaces/Rotational Multibody Interface  Commented=on
  STL Mounting plate : sm_lib/Body Elements/File Solid  Commented=on  ExtGeomFileName=mounting plate.STL  UnitType=Custom  ExtGeomFileUnits=mm  StepReaderType=HEX  ExportConvexHullGeometry=off  InertiaType=Custom  BasedOnType=DensityFromFile  Density=1000  DensityUnits=kg/m^3  Mass=0  MassUnits=kg  CenterOfMass=[0 0 0]  CenterOfMassUnits=m  MomentsOfInertia=[0 0 0]  MomentsOfInertiaUnits=kg*m^2  ProductsOfInertia=[0 0 0]  ProductsOfInertiaUnits=kg*m^2  GraphicType=FromGeometry  MarkerShape=Sphere  MarkerSize=10  GraphicVisPropType=SimpleVisualProperties  GraphicDiffuseColor=[0.502 0.502 0.502]  GraphicOpacity=1  GraphicSpecularColor=[0 1 0]  GraphicAmbientColor=[0 0.4471 0.7412]  GraphicEmissiveColor=[0.05882 1 1]  GraphicShininess=75  DoExposeReferenceFrame=on  SerializedFrames=<Frames/>
  STL Winch : sm_lib/Body Elements/File Solid  Commented=on  ExtGeomFileName=winch.STL  UnitType=Custom  ExtGeomFileUnits=mm  StepReaderType=HEX  ExportConvexHullGeometry=off  InertiaType=Custom  BasedOnType=DensityFromFile  Density=1000  DensityUnits=kg/m^3  Mass=0  MassUnits=kg  CenterOfMass=[0 0 0]  CenterOfMassUnits=m  MomentsOfInertia=[0 0 0]  MomentsOfInertiaUnits=kg*m^2  ProductsOfInertia=[0 0 0]  ProductsOfInertiaUnits=kg*m^2  GraphicType=FromGeometry  MarkerShape=Sphere  MarkerSize=10  GraphicVisPropType=SimpleVisualProperties  GraphicDiffuseColor=[0.502 0.502 0.502]  GraphicOpacity=1  GraphicSpecularColor=[0 1 0]  GraphicAmbientColor=[0 0.4471 0.7412]  GraphicEmissiveColor=[0.05882 1 1]  GraphicShininess=75  DoExposeReferenceFrame=on  SerializedFrames=<Frames/>
  STL visual1 : sm_lib/Body Elements/File Solid  Commented=on  ExtGeomFileName=pulley.STL  UnitType=Custom  ExtGeomFileUnits=mm  StepReaderType=HEX  ExportConvexHullGeometry=off  InertiaType=Custom  BasedOnType=DensityFromFile  Density=1000  DensityUnits=kg/m^3  Mass=0  MassUnits=kg  CenterOfMass=[0 0 0]  CenterOfMassUnits=m  MomentsOfInertia=[0 0 0]  MomentsOfInertiaUnits=kg*m^2  ProductsOfInertia=[0 0 0]  ProductsOfInertiaUnits=kg*m^2  GraphicType=FromGeometry  MarkerShape=Sphere  MarkerSize=10  GraphicVisPropType=SimpleVisualProperties  GraphicDiffuseColor=[0.502 0.502 0.502]  GraphicOpacity=1  GraphicSpecularColor=[0 1 0]  GraphicAmbientColor=[0 0.4471 0.7412]  GraphicEmissiveColor=[0.05882 1 1]  GraphicShininess=75  DoExposeReferenceFrame=on  SerializedFrames=<Frames/>
  Scope : Scope  Commented=on  NumInputPorts=2
  Scope1 : Scope  Commented=on
  Scope2 : Scope  Commented=on
  Subsystem2 : Subsystem  Commented=on
      settings: PortSchema="{\"entries\":[{\"content\":{\"sides\":[{\"content\":{\"connectorIds\":[\"In1\"]},\"type\":\"ConnectorPlacement.EquallySpacedRectSide\",\"uuid\":\"6993dbde-6cba-46a2-b1d5-f1047b136426\"},{\"content\":{\"side\":\"RIGHT\"},\"type\":\"ConnectorPlacement.EquallySpacedRectSide\",\"uuid\":\"3ad9b2a3-36be-44b7-a33f-fa48c865a093\"},{\"content\":{\"connectorIds\":[\"LConn1\",\"LConn2\"],\"side\":\"TOP\"},\"type\":\"ConnectorPlacement.EquallySpacedRectSide\",\"uuid\":\"66e9811c-0a42-4ab5-bd83-e8b75281c572\"},{\"content\":{\"connectorIds\":[\"RConn1\",\"RConn2\"],\"side\":\"BOTTOM\"},\"type\":\"ConnectorPlacement.EquallySpacedRectSide\",\"uuid\":\"046bb913-9a9e-4ef9-939b-8e65f57c81b5\"}]},\"type\":\"ConnectorPlacement.EquallySpacedConnector\",\"uuid\":\"5e1ffb91-7437-41ca-a8e1-7c47f283d11a\"}],\"packageUris\":[\"http://schema.mathworks.com/mf0/Connector/R2020b\"],\"version\":\"1.0\"}"
  Top Pulley Constraint : sm_lib/Belts and Cables/Pulley  Commented=on  PitchRadius=r_P  PitchRadiusUnits=m  InitialWrapAngleLowerBound=0  InitialWrapAngleLowerBoundUnits=deg  SenseWrapAngle=off  SensePulleyAngleA=off  SensePulleyAngleB=off  SenseFleetAngleA=off  SenseFleetAngleB=off
  Winch : sm_lib/Body Elements/Cylindrical Solid  CylinderRadius=r_W  CylinderRadiusUnits=m  CylinderLength=L_W  CylinderLengthUnits=m  ExportEntireGeometry=off  InertiaType=Custom  BasedOnType=Density  Density=1000  DensityUnits=kg/m^3  Mass=1  MassUnits=kg  CenterOfMass=[0 0 0]  CenterOfMassUnits=m  MomentsOfInertia=[1 1 1]  MomentsOfInertiaUnits=kg*m^2  ProductsOfInertia=[0 0 0]  ProductsOfInertiaUnits=kg*m^2  GraphicType=FromGeometry  MarkerShape=Sphere  MarkerSize=10  GraphicVisPropType=SimpleVisualProperties  GraphicDiffuseColor=[0.149 0.149 0.149]  GraphicOpacity=1  GraphicSpecularColor=[0.5 0.5 0.5 1.0]  GraphicAmbientColor=[0.15 0.15 0.15 1.0]  GraphicEmissiveColor=[0.0 0.0 0.0 1.0]  GraphicShininess=75  DoExposeReferenceFrame=on  SerializedFrames=<Frames/>
  Winch_Inertia : sm_lib/Body Elements/Inertia  InertiaType=Custom  Mass=Winch_mass  MassUnits=kg  CenterOfMass=[0,0,0]  CenterOfMassUnits=m  MomentsOfInertia=Winch_MOI  MomentsOfInertiaUnits=kg*m^2  ProductsOfInertia=Winch_POI  ProductsOfInertiaUnits=kg*m^2  GraphicType=Marker  MarkerShape=Sphere  MarkerSize=20  GraphicVisPropType=SimpleVisualProperties  GraphicDiffuseColor=[1 0 1]  GraphicOpacity=1  GraphicSpecularColor=[0.5 0.5 0.5 1.0]  GraphicAmbientColor=[0.15 0.15 0.15 1.0]  GraphicEmissiveColor=[0.0 0.0 0.0 1.0]  GraphicShininess=75
  Winch_mass senter : sm_lib/Frames and Transforms/Rigid Transform  RotationMethod=None  FollAlignAxisA=+X  BaseAlignAxisA=+Y  FollAlignAxisB=+Y  BaseAlignAxisB=+Z  RotationStandardAxis=+Z  RotationAngle=0  RotationAngleUnits=deg  RotationArbitraryAxis=[0 0 1]  RotationSequenceAxes=FollowerAxes  RotationSequence=XYX  RotationSequenceAngles=[0 0 0]  RotationSequenceAnglesUnits=deg  RotationMatrix=[1 0 0;0 1 0;0 0 1]  Quaternion=[1 0 0 0]  TranslationMethod=Cartesian  TranslationCartesianOffset=Winch_COM  TranslationCartesianOffsetUnits=m  TranslationStandardAxis=+Z  TranslationStandardOffset=0  TranslationStandardOffsetUnits=m  TranslationROffset=0  TranslationROffsetUnits=m  TranslationThetaOffset=0  TranslationThetaOffsetUnits=deg  TranslationZOffset=0  TranslationZOffsetUnits=m
  winch pos : PMIOPort  Side=Left
  Winch hyd : PMIOPort  Port=2  Side=Left
  wires:
  PS-Simulink Converter1/1 -> Scope1/1
  PS-Simulink Converter2/1 -> Scope2/1
  Constant/1 -> Subsystem2/1(Ctrl)
  PS-Simulink Converter3/1 -> Scope/1  "Etter"
  PS-Simulink Converter4/1 -> Scope/2  "Før"
  connections:
  PS-Simulink Converter2/LConn1 -- Rotational Multibody Interface1/LConn1 -- Revolute Joint2/LConn2
  winch pos/RConn1 -- Rigid Transform1/LConn1
  Belt-Cable Spool1/RConn1 -- Pulley1/RConn1 -- Cable Properties/LConn1
  Belt-Cable Spool1/LConn1 -- Cylindrical Solid1/RConn1 -- Revolute Joint3/RConn1 -- Winch/RConn1
  Belt-Cable End2/LConn1 -- Planar Joint/RConn1
  Belt-Cable End2/RConn1 -- Top Pulley Constraint/RConn1
  Pulley/RConn1 -- Planar Joint/LConn1 -- Revolute Joint1/RConn1 -- Rigid Transform5/LConn1 -- Top Pulley Constraint/LConn1
  Revolute Joint1/LConn1 -- STL visual1/RConn1 -- Rigid Transform2/RConn1
  Revolute Joint2/RConn2 -- PS-Simulink Converter1/LConn1 -- Rotational Multibody Interface1/RConn1
  Rotational Multibody Interface1/LConn2 -- Ideal Rotational Motion Sensor1/RConn1 -- Planetary Gear/LConn1 -- Ideal Rotational Motion Sensor/RConn1 -- Mechanical Rotational Reference1/LConn1 -- Fixed-Displacement Motor (IL)/RConn2
  Subsystem2/RConn1 -- Winch hyd/RConn1
  Subsystem2/LConn2 -- Fixed-Displacement Motor (IL)/RConn3
  Subsystem2/LConn1 -- Fixed-Displacement Motor (IL)/LConn1
  Reservoir (IL)/LConn1 -- Subsystem2/RConn2
  Inertia/LConn1 -- Planetary Gear/RConn2 -- Ideal Rotational Motion Sensor/LConn1 -- Fixed-Displacement Motor (IL)/RConn1
  Ideal Rotational Motion Sensor1/LConn1 -- Rotational Multibody Interface1/RConn2 -- Planetary Gear/RConn1
  Ideal Rotational Motion Sensor1/RConn2 -- PS-Simulink Converter3/LConn1
  Ideal Rotational Motion Sensor/RConn2 -- PS-Simulink Converter4/LConn1
  Rigid Transform3/RConn1 -- Revolute Joint/RConn1
  Revolute Joint/LConn1 -- Pulley1/LConn1 -- Cylindrical Solid/RConn1
  Pulley1/RConn2 -- Top Pulley Constraint/RConn2
  STL Mounting plate/RConn1 -- Rigid Transform4/LConn1
  Winch_Inertia/RConn1 -- Winch_mass senter/RConn1
  STL Winch/RConn1 -- Winch_mass senter/LConn1 -- Rigid Transform1/RConn1 -- Rigid Transform2/LConn1 -- Rigid Transform3/LConn1 -- Revolute Joint3/LConn1 -- Rigid Transform4/RConn1
  Brick Solid/RConn1 -- Rigid Transform5/RConn1 -- Rigid Transform6/LConn1
  Rigid Transform7/LConn1 -- Rigid Transform6/RConn1
  Load/RConn1 -- Rigid Transform7/RConn1

== system RedCrane_Control_System_17032025/Jib cylinder/Subsystem ==
  PA_JibC : Gain  Gain=1/1e5
  PS-Simulink Converter2 : nesl_utility/PS-Simulink Converter  PhysicalDomain=network_engine_domain  SubClassName=ps_output  LeftPortType=input  RightPortType=output  PseudoPeriodic=off  Frequencies=[]  VectorFormat=inherit  Unit=inherit  AffineConversion=off
  Pressure Sensor (IL) : fl_lib/Isothermal Liquid/Sensors/Pressure Sensor (IL)  pressure_measure=foundation.enum.pressure_measure.gauge
      settings: InternalSimscapePortConfiguration="{\"Bottom\":[],\"Left\":[{\"id\":\"A\",\"label\":\"A\",\"type\":\"foundation.isothermal_liquid.isothermal_liquid\"}],\"Right\":[{\"id\":\"Pg\",\"label\":\"Pg\",\"type\":\"output\"}],\"Top\":[]}"
  Scope2 : Scope
  Conn1 : PMIOPort  Side=Right
  wires:
  PS-Simulink Converter2/1 -> PA_JibC/1
  PA_JibC/1 -> Scope2/1
  connections:
  PS-Simulink Converter2/LConn1 -- Pressure Sensor (IL)/RConn1
  Pressure Sensor (IL)/LConn1 -- Conn1/RConn1

== system RedCrane_Control_System_17032025/Jib cylinder/Subsystem1 ==
  PB_JibC : Gain  Gain=1/1e5
  PS-Simulink Converter2 : nesl_utility/PS-Simulink Converter  PhysicalDomain=network_engine_domain  SubClassName=ps_output  LeftPortType=input  RightPortType=output  PseudoPeriodic=off  Frequencies=[]  VectorFormat=inherit  Unit=inherit  AffineConversion=off
  Pressure Sensor (IL) : fl_lib/Isothermal Liquid/Sensors/Pressure Sensor (IL)  pressure_measure=foundation.enum.pressure_measure.gauge
      settings: InternalSimscapePortConfiguration="{\"Bottom\":[],\"Left\":[{\"id\":\"A\",\"label\":\"A\",\"type\":\"foundation.isothermal_liquid.isothermal_liquid\"}],\"Right\":[{\"id\":\"Pg\",\"label\":\"Pg\",\"type\":\"output\"}],\"Top\":[]}"
  Scope2 : Scope
  Conn1 : PMIOPort  Side=Right
  wires:
  PS-Simulink Converter2/1 -> PB_JibC/1
  PB_JibC/1 -> Scope2/1
  connections:
  PS-Simulink Converter2/LConn1 -- Pressure Sensor (IL)/RConn1
  Pressure Sensor (IL)/LConn1 -- Conn1/RConn1
